simulink model "suspension_system_Model"  (R2020a)
settings: Solver=VariableStepAuto  StartTime=0.0  StopTime=10.0  RelTol=1e-3
undefined symbols (not defined in the file): b, k1, k2, m1, m2, x
settings Model: Creator=INDRAJIT MARATHE  LastModifiedBy=INDRAJIT MARATHE

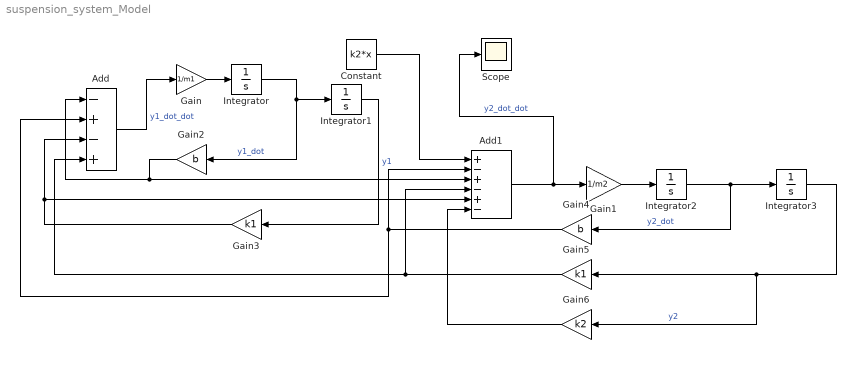
== system suspension_system_Model ==
  Add : Sum  Inputs=-+-+
  Add1 : Sum  Inputs=+-+-+-
  Constant : Constant  Value=k2*x
  Gain : Gain  Gain=1/m1
  Gain1 : Gain  Gain=1/m2
  Gain2 : Gain  Gain=b
  Gain3 : Gain  Gain=k1
  Gain4 : Gain  Gain=b
  Gain5 : Gain  Gain=k1
  Gain6 : Gain  Gain=k2
  Integrator{,1..3} (4 alike) : Integrator
  Scope : Scope
  wires:
  Add1/1 -> Scope/1, Gain1/1  "y2_dot_dot"
  Add/1 -> Gain/1  "y1_dot_dot"
  Integrator/1 -> Gain2/1, Integrator1/1  "y1_dot"
  Integrator2/1 -> Gain4/1, Integrator3/1  "y2_dot"
  Gain/1 -> Integrator/1
  Gain1/1 -> Integrator2/1
  Integrator3/1 -> Gain6/1, Gain5/1  "y2"
  Integrator1/1 -> Gain3/1  "y1"
  Gain2/1 -> Add/1, Add1/3
  Gain3/1 -> Add/3, Add1/5
  Gain4/1 -> Add/2, Add1/2
  Gain5/1 -> Add/4, Add1/4
  Gain6/1 -> Add1/6
  Constant/1 -> Add1/1
